simulink model "quadrotor_PID_controllers"  (R2021a)
settings: Solver=FixedStepAuto  StartTime=0.0  StopTime=10.0  FixedStep=1/sim_freq  RelTol=1e-3
undefined symbols (not defined in the file): max_tilt, mpc_start_time, payload_angle_ref, sim_freq, thr_max, thr_min, u_bar
libraries: mpclib x1
settings Model: Creator=francois  LastModifiedBy=esl
settings SolverCC: AlgebraicLoopSolver=TrustRegion
settings DebuggingCC: SFMachineParentedDataDiag=warning
settings ModelReferenceCC: ModelReferenceNumInstancesAllowed=Single

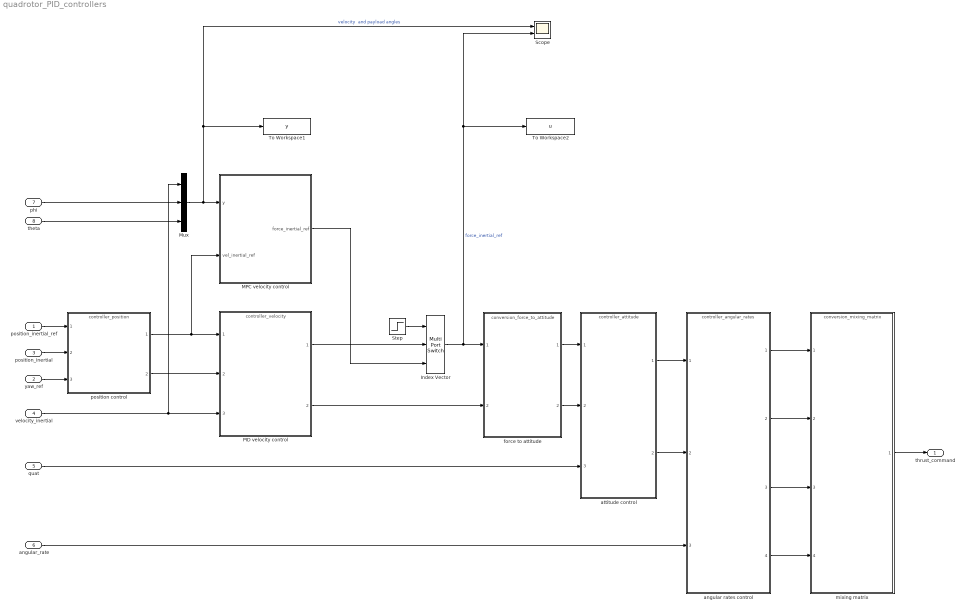
== system quadrotor_PID_controllers ==
  position_inertial_ref : Inport
  yaw_ref : Inport  Port=2
  position_inertial : Inport  Port=3
  velocity_inertial : Inport  Port=4
  quat : Inport  Port=5  PortDimensions=4
  angular_rate : Inport  Port=6
  phi : Inport  Port=7
  theta : Inport  Port=8
  Index Vector : MultiPortSwitch  DataPortOrder=Zero-based contiguous  Inputs=2  zeroidx=on
  MPC velocity control : Subsystem
  Mux : Mux  Inputs=3
  PID velocity control : ModelReference  ModelNameDialog=controller_velocity.slx  SimulationMode=Normal  ModelReferenceVersion=3.0
  Scope : Scope  NumInputPorts=2
  Step : Step  Time=mpc_start_time  SampleTime=0
  To Workspace1 : ToWorkspace  VariableName=y  SaveFormat=Timeseries  SampleTime=-1
  To Workspace2 : ToWorkspace  VariableName=u  SaveFormat=Timeseries  SampleTime=-1
  angular rates control : ModelReference  ModelNameDialog=controller_angular_rates.slx  SimulationMode=Normal  ModelReferenceVersion=3.0
  attitude control : ModelReference  ModelNameDialog=controller_attitude.slx  SimulationMode=Normal  ModelReferenceVersion=3.0
  force to attitude : ModelReference  ModelNameDialog=conversion_force_to_attitude.slx  SimulationMode=Normal  ModelReferenceVersion=1.7
  mixing matrix : ModelReference  ModelNameDialog=conversion_mixing_matrix.slx  SimulationMode=Normal  ModelReferenceVersion=1.7
  position control : ModelReference  ModelNameDialog=controller_position.slx  SimulationMode=Normal  ModelReferenceVersion=4.0
  thrust_command : Outport
  wires:
  position control/2 -> PID velocity control/2
  angular rates control/3 -> mixing matrix/3
  angular_rate/1 -> angular rates control/3
  quat/1 -> attitude control/3
  angular rates control/1 -> mixing matrix/1
  angular rates control/4 -> mixing matrix/4
  mixing matrix/1 -> thrust_command/1
  attitude control/1 -> angular rates control/1
  velocity_inertial/1 -> Mux/1, PID velocity control/3
  position_inertial/1 -> position control/2
  angular rates control/2 -> mixing matrix/2
  force to attitude/2 -> attitude control/2
  attitude control/2 -> angular rates control/2
  yaw_ref/1 -> position control/3
  position_inertial_ref/1 -> position control/1
  force to attitude/1 -> attitude control/1
  PID velocity control/2 -> force to attitude/2
  position control/1 -> MPC velocity control/2(vel_inertial_ref), PID velocity control/1
  PID velocity control/1 -> Index Vector/2
  MPC velocity control/1(force_inertial_ref) -> Index Vector/3
  Step/1 -> Index Vector/1
  Index Vector/1 -> Scope/2, To Workspace2/1, force to attitude/1  "force_inertial_ref"
  phi/1 -> Mux/2
  theta/1 -> Mux/3
  Mux/1 -> Scope/1, To Workspace1/1, MPC velocity control/1(y)  "velocity  and payload angles"

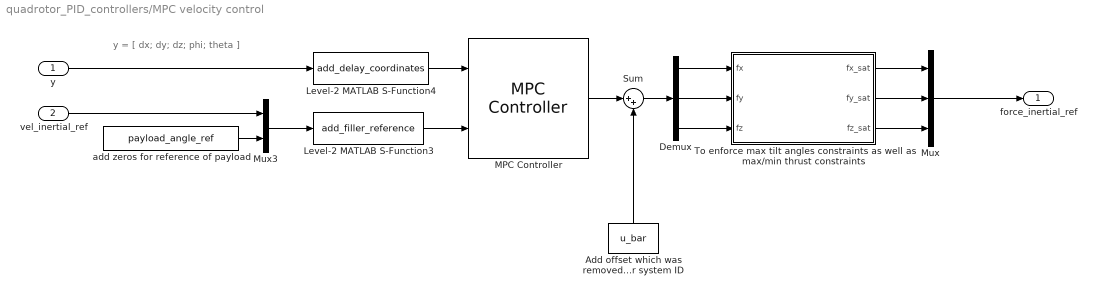
== system quadrotor_PID_controllers/MPC velocity control ==
  note: y = [ dx; dy; dz; phi; theta ]
  y : Inport
  vel_inertial_ref : Inport  Port=2
  Add offset which was removed for system ID : Constant  Value=u_bar
  Demux : Demux  Outputs=3
  Level-2 MATLAB S-Function3 : M-S-Function  FunctionName=add_filler_reference  Parameters=ny, q, Ts_mpc
  Level-2 MATLAB S-Function4 : M-S-Function  FunctionName=add_delay_coordinates  Parameters=y_ext_0, q, Ts_mpc, ny
  MPC Controller : mpclib/MPC Controller  SCDEnableBlockLinearizationSpecification=on  mpcobj=mpc_vel  is_multiple=0  enable_value=0  return_u0=off  updateMPCinCallerWorkspace=on  md_inport=off  mv_inport=off  uref_inport=off  return_cost=off  return_mvseq=off  return_qpstatus=off  return_xseq=off  return_state=off  return_ovseq=off  state_inport=off  umin_inport=off  umax_inport=off  ymin_inport=off  ymax_inport=off  cc_inport=off  ywt_inport=off  uwt_inport=off  duwt_inport=off  rhoeps_inport=off  pm_inport=off  MaximumP=10  HorizonChoice=FixedHorizon  n_ts=0.03  n_p=200  n_mv=3  n_md=0  n_ud=0  n_mo=30  n_uo=0  BlockDataType=double  SampleTimeInherited=off  switch_inport=off
  Mux : Mux  Inputs=3
  Mux3 : Mux  Inputs=2
  Sum : Sum  Inputs=|++
  To enforce max tilt angles constraints as well as max/min thrust constraints : MATLAB Function  TreatAsAtomicUnit=on  SystemSampleTime=1/sim_freq
  add zeros for reference of payload : Constant  Value=payload_angle_ref
  force_inertial_ref : Outport
  wires:
  Level-2 MATLAB S-Function3/1 -> MPC Controller/2
  Level-2 MATLAB S-Function4/1 -> MPC Controller/1
  To enforce max tilt angles constraints as well as max/min thrust constraints/3(fz_sat) -> Mux/3
  To enforce max tilt angles constraints as well as max/min thrust constraints/1(fx_sat) -> Mux/1
  To enforce max tilt angles constraints as well as max/min thrust constraints/2(fy_sat) -> Mux/2
  Demux/2 -> To enforce max tilt angles constraints as well as max/min thrust constraints/2(fy)
  Demux/3 -> To enforce max tilt angles constraints as well as max/min thrust constraints/3(fz)
  Demux/1 -> To enforce max tilt angles constraints as well as max/min thrust constraints/1(fx)
  Mux/1 -> force_inertial_ref/1
  MPC Controller/1 -> Sum/1
  Sum/1 -> Demux/1
  Add offset which was removed for system ID/1 -> Sum/2
  Mux3/1 -> Level-2 MATLAB S-Function3/1
  add zeros for reference of payload/1 -> Mux3/2
  vel_inertial_ref/1 -> Mux3/1
  y/1 -> Level-2 MATLAB S-Function4/1

== matlab function quadrotor_PID_controllers/MPC velocity control/To enforce max tilt angles constraints as well as max//min thrust constraints ==
  data: fx input; fx_sat output; fy input; fz input; fy_sat output; max_tilt parameter; thr_max parameter; fz_sat output; thr_min parameter
function [fx_sat, fy_sat, fz_sat] = constrain_max_tilt(fx, fy, fz, max_tilt, thr_max, thr_min)
    % First constrain fz.
    if fz > -thr_min
        fz_sat = -thr_min;
    elseif fz < -thr_max
        fz_sat = -thr_max;
    else
        fz_sat = fz;
    end
    
    % Constrain fx and fy
    thrust_max_NE_tilt = abs(fz_sat) * tan(max_tilt * pi/180);
    thrust_max_NE = sqrt(thr_max*thr_max - fz_sat*fz_sat);
    thrust_max_NE = min(thrust_max_NE_tilt, thrust_max_NE);
    
    fx_sat = fx;
    fy_sat = fy;

%     if dot([fx, fy], [fx, fy]) > thrust_max_NE*thrust_max_NE
%         mag = norm([fx, fy]);
    mag = norm([fx, fy]); %myne
    if mag > thrust_max_NE% myne
        fx_sat = fx / mag * thrust_max_NE;
        fy_sat = fy / mag * thrust_max_NE;
    end
end
